simulink model "sim_1"  (R2015b)
settings: Solver=ode23  StartTime=0  StopTime=tstop  FixedStep=1e-3  RelTol=1e-4
undefined symbols (not defined in the file or in its folder): alpha_nc, alpha_nw, currentCoeffMatrix, f, mu, N_freq, Par, phi, S, Sim, U_mean_c, U_mean_w, windCoeffMatrix
libraries: simulink_extras x4, simulink x4
settings Model: Creator=torstebo  LastModifiedBy=ShivJeet
settings SolverCC: MaxConsecutiveMinStep=3  SolverJacobianMethodControl=FullPerturbation  ZeroCrossControl=DisableAll  ZeroCrossAlgorithm=Adaptive
settings DataIOCC: Decimation=10  InitialState=xFinal  LimitDataPoints=off  SaveFormat=StructureWithTime  SaveOutput=off  InspectSignalLogs=on  VisualizeSimOutput=off  SaveTime=off
settings OptimizationCC: AccelVerboseBuild=on
settings DebuggingCC: AlgebraicLoopMsg=error  UnderspecifiedInitializationDetection=Classic  MergeDetectMultiDrivingBlocksExec=none  SolverPrmCheckMsg=warning  StateNameClashWarn=warning
settings HardwareCC: ProdBitPerPointer=32  ProdLargestAtomicFloat=None  ProdIntDivRoundTo=Undefined  ProdEndianess=Unspecified  ProdWordSize=32  ProdHWDeviceType=32-bit Generic
settings GRTTargetCC: GeneratePreprocessorConditionals=Disable all
settings ConfigComp: CovModelRefEnable=Off  CovSFcnEnable=off

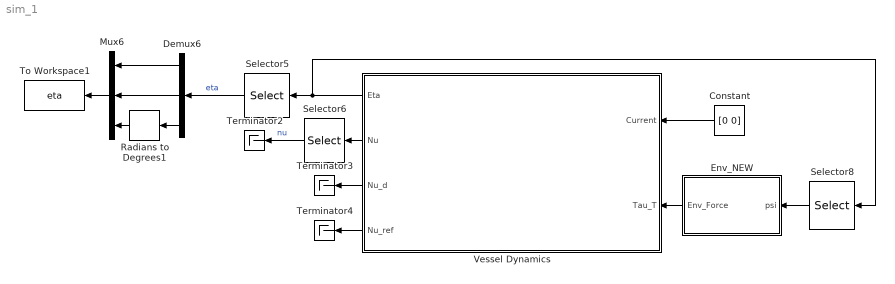
== system sim_1 ==
  Constant : Constant  Value=[0 0]
  Demux6 : Demux  Outputs=3
  Env_NEW : Subsystem
  Mux6 : Mux  Inputs=3
  Radians to Degrees1 : simulink_extras/Transformations/Radians to Degrees
  Selector5 : Selector  InputPortWidth=6  IndexOptions=Index vector (dialog)  Indices=[1 2 6]  OutputSizes=1
  Selector6 : Selector  InputPortWidth=6  IndexOptions=Index vector (dialog)  Indices=[1 2 6]  OutputSizes=1
  Selector8 : Selector  InputPortWidth=6  IndexOptions=Index vector (dialog)  Indices=[6]  OutputSizes=1
  Terminator2 : Terminator
  Terminator3 : Terminator
  Terminator4 : Terminator
  To Workspace1 : ToWorkspace  VariableName=eta  SaveFormat=Timeseries  SampleTime=-1
  Vessel Dynamics : Subsystem
      mask Display:
      | image(imread('Files/supply.jpg'))
      | color('black'); port_label('output', 1, 'eta')
      | color('black'); port_label('output', 2, 'nu')
      | color('black'); port_label('output', 3, 'nu_d')
      | color('black'); port_label('output', 4, 'nu_ref')
      | color('black'); port_label('input', 1, 'nu_c')
      | color('black'); port_label('input', 2, 'tau')
  wires:
  Vessel Dynamics/1(Eta) -> Selector8/1, Selector5/1
  Vessel Dynamics/2(Nu) -> Selector6/1
  Constant/1 -> Vessel Dynamics/1(Current)
  Env_NEW/1(Env_Force) -> Vessel Dynamics/2(Tau_T)
  Selector8/1 -> Env_NEW/1(psi)
  Vessel Dynamics/3(Nu_d) -> Terminator3/1
  Vessel Dynamics/4(Nu_ref) -> Terminator4/1
  Selector5/1 -> Demux6/1  "eta"
  Demux6/3 -> Radians to Degrees1/1
  Radians to Degrees1/1 -> Mux6/3
  Demux6/2 -> Mux6/2
  Demux6/1 -> Mux6/1
  Mux6/1 -> To Workspace1/1
  Selector6/1 -> Terminator2/1  "nu"

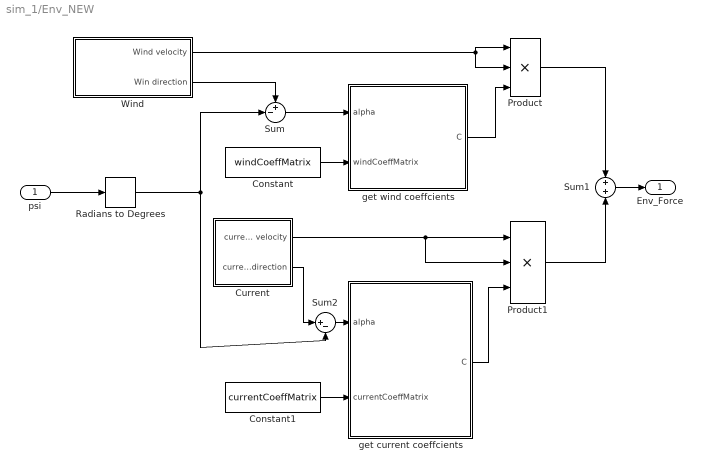
== system sim_1/Env_NEW ==
  psi : Inport
  Constant : Constant  Value=windCoeffMatrix
  Constant1 : Constant  Value=currentCoeffMatrix
  Current : Subsystem
  Product : Product  Inputs=3  RndMeth=Zero
  Product1 : Product  Inputs=3  RndMeth=Zero
  Radians to Degrees : simulink_extras/Transformations/Radians to Degrees
  Sum : Sum  Inputs=+-|
  Sum1 : Sum  Inputs=+|+
  Sum2 : Sum  Inputs=|+-
  Wind : Subsystem
  get current coeffcients : MATLAB Function  TreatAsAtomicUnit=on
  get wind coeffcients : MATLAB Function  TreatAsAtomicUnit=on
  Env_Force : Outport
  wires:
  Wind/1(Wind velocity) -> Product/2, Product/1
  Wind/2(Win direction) -> Sum/1
  psi/1 -> Radians to Degrees/1
  Sum1/1 -> Env_Force/1
  Current/1(current velocity) -> Product1/2, Product1/1
  Radians to Degrees/1 -> Sum/2, Sum2/2
  Current/2(current direction) -> Sum2/1
  Sum2/1 -> get current coeffcients/1(alpha)
  get current coeffcients/1(C) -> Product1/3
  Sum/1 -> get wind coeffcients/1(alpha)
  get wind coeffcients/1(C) -> Product/3
  Product1/1 -> Sum1/2
  Product/1 -> Sum1/1
  Constant/1 -> get wind coeffcients/2(windCoeffMatrix)
  Constant1/1 -> get current coeffcients/2(currentCoeffMatrix)

== system sim_1/Vessel Dynamics ==
  note: VESSEL MODULE
      | Consists of a WF and a LF module, which may be enabled or disabled in the Parameters file.
      | The LF and WFmotion components are written to the workspace for processing, and added for
      | use in the simulator.
  Current : Inport
  Tau_T : Inport  Port=2
  Vessel LF 6DOF : Subsystem
  Eta : Outport
  Nu : Outport  Port=2
  Nu_d : Outport  Port=3
  Nu_ref : Outport  Port=4
  wires:
  Current/1 -> Vessel LF 6DOF/2(Current_NED)
  Tau_T/1 -> Vessel LF 6DOF/1(External forces)  "Tau_T"
  Vessel LF 6DOF/1(Eta) -> Eta/1  "Eta_LF"
  Vessel LF 6DOF/2(Nu) -> Nu/1  "Nu_LF"
  Vessel LF 6DOF/3(Nu_d) -> Nu_d/1
  Vessel LF 6DOF/4(Nu_r) -> Nu_ref/1

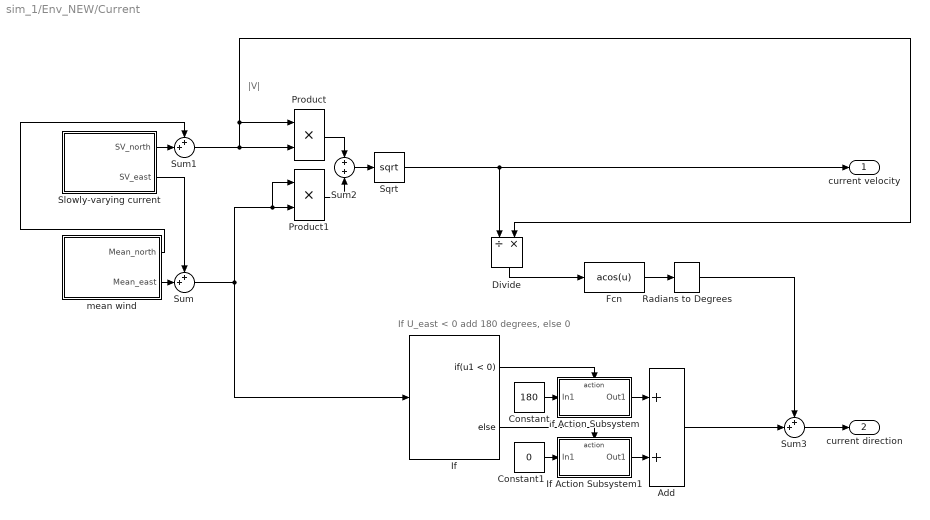
== system sim_1/Env_NEW/Current ==
  note: If U_east < 0 add 180 degrees, else 0
  note: |V|
  Add : Sum
  Constant : Constant  Value=180
  Constant1 : Constant  Value=0
  Divide : Product  Inputs=/*
  Fcn : Fcn  Expr=acos(u)
  "If " : If  IfExpression=u1 < 0
  If Action Subsystem : Subsystem  TreatAsAtomicUnit=on
  If Action Subsystem1 : Subsystem  TreatAsAtomicUnit=on
  Product : Product
  Product1 : Product
  Radians to Degrees : simulink_extras/Transformations/Radians to Degrees
  Slowly-varying current : Subsystem
  Sqrt : Sqrt  SaturateOnIntegerOverflow=on
  Sum : Sum  Inputs=++|
  Sum1 : Sum  Inputs=++|
  Sum2 : Sum  Inputs=+|+
  Sum3 : Sum  Inputs=++|
  mean wind : Subsystem
  current velocity : Outport
  current direction : Outport  Port=2
  wires:
  Slowly-varying current/1(SV_north) -> Sum1/2
  Slowly-varying current/2(SV_east) -> Sum/1
  mean wind/2(Mean_east) -> Sum/2
  Divide/1 -> Fcn/1
  Fcn/1 -> Radians to Degrees/1
  Sum3/1 -> current direction/1
  Radians to Degrees/1 -> Sum3/1
  If Action Subsystem/1(Out1) -> Add/1
  Add/1 -> Sum3/2
  mean wind/1(Mean_north) -> Sum1/1
  Sum1/1 -> Product/2, Product/1, Divide/2
  Sum/1 -> Product1/1, Product1/2, "If "/1
  Product/1 -> Sum2/1
  Product1/1 -> Sum2/2
  Sum2/1 -> Sqrt/1
  Sqrt/1 -> Divide/1, current velocity/1
  Constant/1 -> If Action Subsystem/1(In1)
  "If "/1 -> If Action Subsystem/Action
  "If "/2 -> If Action Subsystem1/Action
  Constant1/1 -> If Action Subsystem1/1(In1)
  If Action Subsystem1/1(Out1) -> Add/2

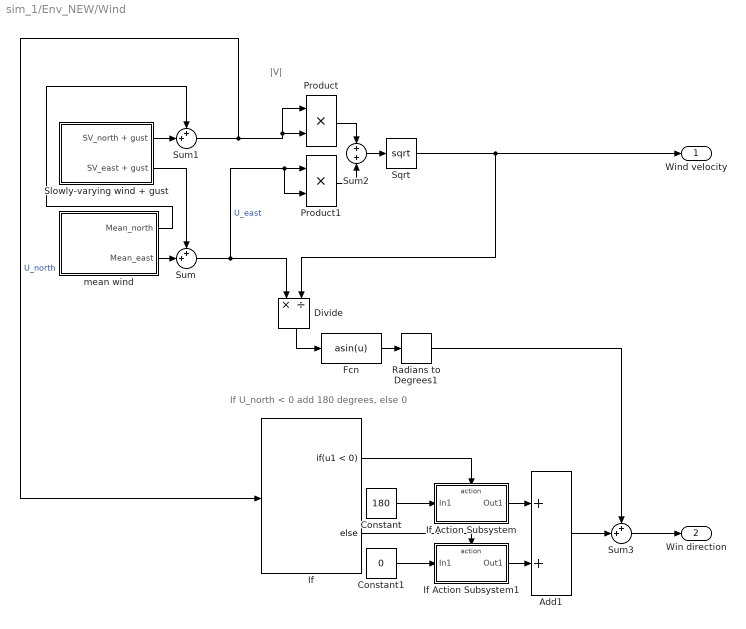
== system sim_1/Env_NEW/Wind ==
  note: |V|
  note: If U_north < 0 add 180 degrees, else 0
  Add1 : Sum
  Constant : Constant  Value=180
  Constant1 : Constant  Value=0
  Divide : Product  Inputs=*/
  Fcn : Fcn  Expr=asin(u)
  If : If  IfExpression=u1 < 0
  If Action Subsystem : Subsystem  TreatAsAtomicUnit=on
  If Action Subsystem1 : Subsystem  TreatAsAtomicUnit=on
  Product : Product
  Product1 : Product
  Radians to Degrees1 : simulink_extras/Transformations/Radians to Degrees
  Slowly-varying wind + gust : Subsystem
  Sqrt : Sqrt  SaturateOnIntegerOverflow=on
  Sum : Sum  Inputs=++|
  Sum1 : Sum  Inputs=++|
  Sum2 : Sum  Inputs=+|+
  Sum3 : Sum  Inputs=++|
  mean wind : Subsystem
  Wind velocity : Outport
  Win direction : Outport  Port=2
  wires:
  Slowly-varying wind + gust/2(SV_east + gust) -> Sum/1
  mean wind/2(Mean_east) -> Sum/2
  Sum1/1 -> Product/1, Product/2, If/1  "U_north"
  Sum/1 -> Product1/2, Product1/1, Divide/1  "U_east"
  Sqrt/1 -> Divide/2, Wind velocity/1
  Slowly-varying wind + gust/1(SV_north + gust) -> Sum1/2
  mean wind/1(Mean_north) -> Sum1/1
  Product/1 -> Sum2/1
  Product1/1 -> Sum2/2
  Sum2/1 -> Sqrt/1
  Divide/1 -> Fcn/1
  Fcn/1 -> Radians to Degrees1/1
  Radians to Degrees1/1 -> Sum3/1
  Add1/1 -> Sum3/2
  Sum3/1 -> Win direction/1
  If Action Subsystem/1(Out1) -> Add1/1
  Constant/1 -> If Action Subsystem/1(In1)
  If/1 -> If Action Subsystem/Action
  If/2 -> If Action Subsystem1/Action
  Constant1/1 -> If Action Subsystem1/1(In1)
  If Action Subsystem1/1(Out1) -> Add1/2

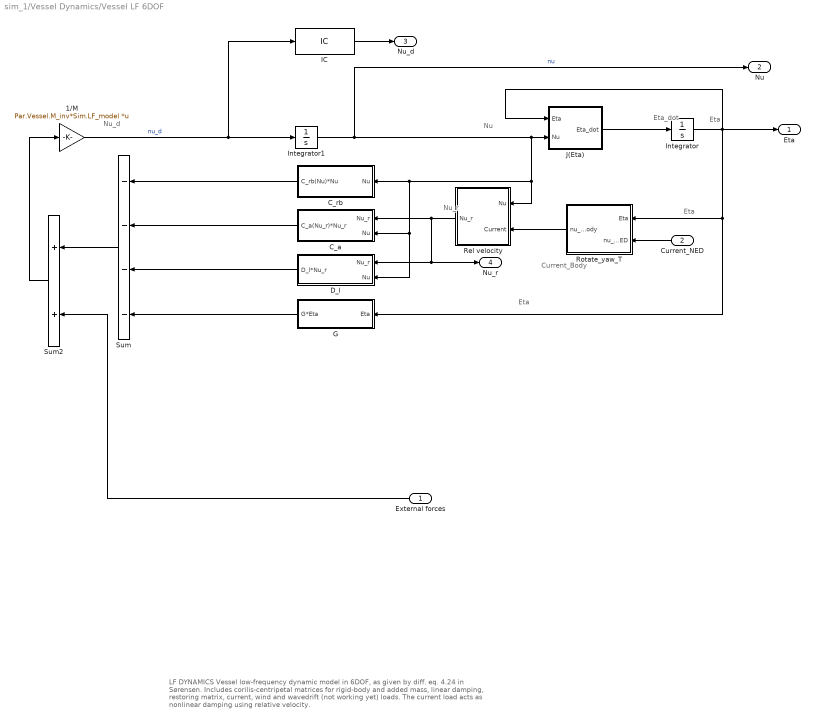
== system sim_1/Vessel Dynamics/Vessel LF 6DOF ==
  note: Nu_d
  note: Nu
  note: Eta
  note: Current_Body
  note: Eta
  note: Nu_r
  note: Eta
  note: LF DYNAMICS
      | Vessel low-frequency dynamic model in 6DOF, as given by diff. eq. 4.24 in Sørensen.
      | Includes corilis-centripetal matrices for rigid-body and added mass, linear damping,
      | restoring matrix, current, wind and wavedrift (not working yet) loads. The current load
      | acts as nonlinear damping using relative velocity.
  note: Eta_dot
  External forces : Inport
  Current_NED : Inport  Port=2
  1/M : Gain  Gain=Par.Vessel.M_inv*Sim.LF_model  Multiplication=Matrix(K*u) (u vector)  SaturateOnIntegerOverflow=on  OutDataTypeStr=Inherit: Same as input  ParamDataTypeStr=Inherit: Same as input
  C_a : Subsystem
  C_rb : Subsystem
  D_l : Subsystem
      settings: MinAlgLoopOccurrences=on
  G : Subsystem
  IC : InitialCondition  Value=Sim.Nu_d_init
  Integrator : Integrator  InitialCondition=Sim.Eta_init
  Integrator1 : Integrator  InitialCondition=Sim.Nu_init
  J(Eta) : Subsystem
  Rel velocity : Subsystem
  Rotate_yaw_T : Subsystem
  Sum : Sum  Inputs=----  SaturateOnIntegerOverflow=on
  Sum2 : Sum  SaturateOnIntegerOverflow=on
  Eta : Outport
  Nu : Outport  Port=2
  Nu_d : Outport  Port=3
  Nu_r : Outport  Port=4
  wires:
  1/M/1 -> IC/1, Integrator1/1  "nu_d"
  J(Eta)/1(Eta_dot) -> Integrator/1
  Integrator/1 -> J(Eta)/1(Eta), Eta/1, Rotate_yaw_T/1(Eta), G/1(Eta)
  Integrator1/1 -> Nu/1, J(Eta)/2(Nu), Rel velocity/1(Nu), C_a/2(Nu), D_l/2(Nu), C_rb/1(Nu)  "nu"
  Current_NED/1 -> Rotate_yaw_T/2(nu_2D_NED)
  Rotate_yaw_T/1(nu_2D_body) -> Rel velocity/2(Current)
  Rel velocity/1(Nu_r) -> D_l/1(Nu_r), Nu_r/1, C_a/1(Nu_r)
  Sum/1 -> Sum2/1
  External forces/1 -> Sum2/2
  Sum2/1 -> 1/M/1
  C_rb/1(C_rb(Nu)*Nu) -> Sum/1
  C_a/1(C_a(Nu_r)*Nu_r) -> Sum/2
  D_l/1(D_l*Nu_r) -> Sum/3
  G/1(G*Eta) -> Sum/4
  IC/1 -> Nu_d/1

== system sim_1/Env_NEW/Current/If Action Subsystem ==
  In1 : Inport
  Action Port : ActionPort  ActionType=then
  Out1 : Outport
  wires:
  In1/1 -> Out1/1

== system sim_1/Env_NEW/Current/If Action Subsystem1 ==
  In1 : Inport
  Action Port : ActionPort  ActionType=else
  Out1 : Outport
  wires:
  In1/1 -> Out1/1

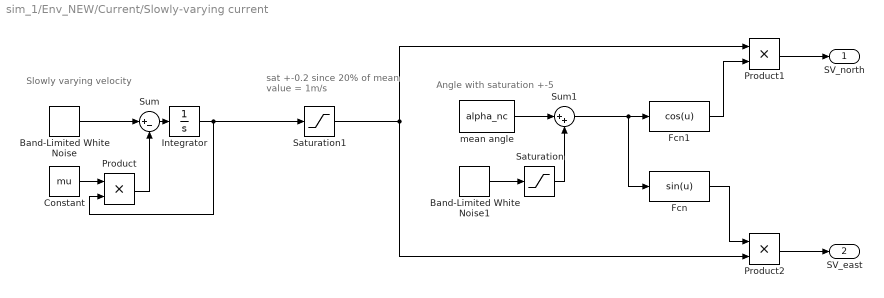
== system sim_1/Env_NEW/Current/Slowly-varying current ==
  note: Angle with saturation +-5
  note: Slowly varying velocity
  note: sat +-0.2 since 20%
      | of mean value = 1m/s
  Band-Limited White Noise : simulink/Sources/Band-Limited White Noise  Cov=[0.00005]  Ts=20  seed=[23343]
  Band-Limited White Noise1 : simulink/Sources/Band-Limited White Noise  Cov=[0.00005]  Ts=20  seed=[23344]
  Constant : Constant  Value=mu
  Fcn : Fcn  Expr=sin(u)
  Fcn1 : Fcn  Expr=cos(u)
  Integrator : Integrator
  Product : Product  RndMeth=Zero
  Product1 : Product  RndMeth=Zero
  Product2 : Product  RndMeth=Zero
  Saturation : Saturate  UpperLimit=(5*pi)/180  LowerLimit=-(5*pi)/180
  Saturation1 : Saturate  UpperLimit=0.2  LowerLimit=-0.2
  Sum : Sum  Inputs=|+-
  Sum1 : Sum  Inputs=|++
  mean angle : Constant  Value=alpha_nc
  SV_north : Outport
  SV_east : Outport  Port=2
  wires:
  Band-Limited White Noise/1 -> Sum/1
  Sum/1 -> Integrator/1
  Integrator/1 -> Product/2, Saturation1/1
  Product/1 -> Sum/2
  Constant/1 -> Product/1
  Fcn1/1 -> Product1/2
  mean angle/1 -> Sum1/1
  Sum1/1 -> Fcn/1, Fcn1/1
  Saturation/1 -> Sum1/2
  Band-Limited White Noise1/1 -> Saturation/1
  Product1/1 -> SV_north/1
  Product2/1 -> SV_east/1
  Saturation1/1 -> Product2/2, Product1/1
  Fcn/1 -> Product2/1

== system sim_1/Env_NEW/Current/mean wind ==
  Constant : Constant  Value=U_mean_c
  Fcn : Fcn  Expr=sin(u)
  Fcn1 : Fcn  Expr=cos(u)
  Product1 : Product  RndMeth=Zero
  Product2 : Product  RndMeth=Zero
  meen wind : Constant  Value=alpha_nc
  Mean_north : Outport
  Mean_east : Outport  Port=2
  wires:
  Constant/1 -> Product1/1, Product2/2
  Fcn1/1 -> Product1/2
  Product1/1 -> Mean_north/1
  Product2/1 -> Mean_east/1
  meen wind/1 -> Fcn/1, Fcn1/1
  Fcn/1 -> Product2/1

== system sim_1/Env_NEW/Wind/If Action Subsystem ==
  In1 : Inport
  Action Port : ActionPort  ActionType=then
  Out1 : Outport
  wires:
  In1/1 -> Out1/1

== system sim_1/Env_NEW/Wind/If Action Subsystem1 ==
  In1 : Inport
  Action Port : ActionPort  ActionType=else
  Out1 : Outport
  wires:
  In1/1 -> Out1/1

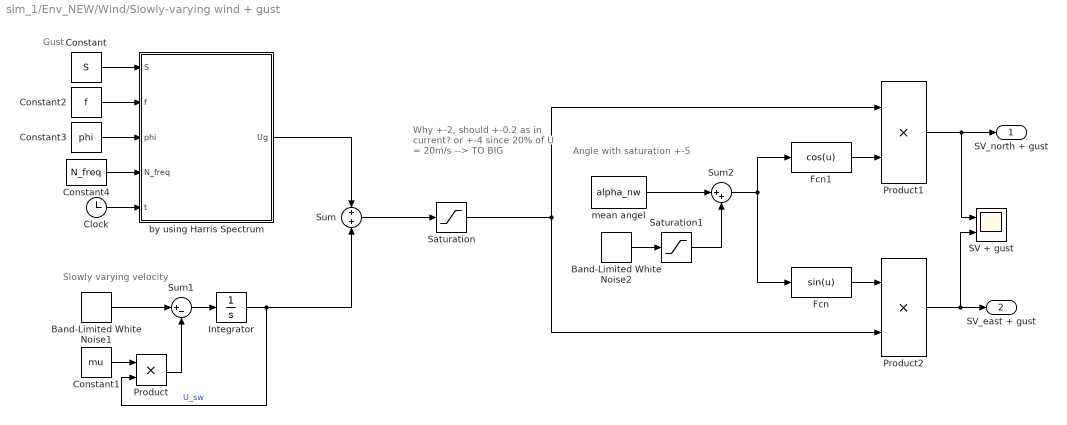
== system sim_1/Env_NEW/Wind/Slowly-varying wind + gust ==
  note: Gust
  note: Slowly varying velocity
  note: Angle with saturation +-5
  note: Why +-2, should
      | +-0.2 as in current?
      | or +-4 since 20% of
      | U = 20m/s --> TO BIG
  Band-Limited White Noise1 : simulink/Sources/Band-Limited White Noise  Cov=[0.005]  Ts=20  seed=[23341]
  Band-Limited White Noise2 : simulink/Sources/Band-Limited White Noise  Cov=[0.005]  Ts=20  seed=[23342]
  Clock : Clock
  Constant : Constant  Value=S
  Constant1 : Constant  Value=mu
  Constant2 : Constant  Value=f
  Constant3 : Constant  Value=phi
  Constant4 : Constant  Value=N_freq
  Fcn : Fcn  Expr=sin(u)
  Fcn1 : Fcn  Expr=cos(u)
  Integrator : Integrator
  Product : Product  RndMeth=Zero
  Product1 : Product  RndMeth=Zero
  Product2 : Product  RndMeth=Zero
  SV + gust : Scope  NumInputPorts=2
  Saturation : Saturate  UpperLimit=2  LowerLimit=-2
  Saturation1 : Saturate  UpperLimit=(5*pi)/180  LowerLimit=-(5*pi)/180
  Sum : Sum  Inputs=+|+
  Sum1 : Sum  Inputs=|+-
  Sum2 : Sum  Inputs=|++
  by using Harris Spectrum : MATLAB Function  TreatAsAtomicUnit=on  SystemSampleTime=1
  mean angel : Constant  Value=alpha_nw
  SV_north + gust : Outport
  SV_east + gust : Outport  Port=2
  wires:
  Fcn1/1 -> Product1/2
  Product1/1 -> SV + gust/1, SV_north + gust/1
  Product2/1 -> SV_east + gust/1, SV + gust/2
  Sum2/1 -> Fcn/1, Fcn1/1
  Integrator/1 -> Sum/2, Product/2  "U_sw"
  Saturation/1 -> Product1/1, Product2/2
  Constant1/1 -> Product/1
  Sum1/1 -> Integrator/1
  Product/1 -> Sum1/2
  Band-Limited White Noise1/1 -> Sum1/1
  mean angel/1 -> Sum2/1
  Saturation1/1 -> Sum2/2
  Band-Limited White Noise2/1 -> Saturation1/1
  Fcn/1 -> Product2/1
  Constant/1 -> by using Harris Spectrum/1(S)
  Constant2/1 -> by using Harris Spectrum/2(f)
  Constant3/1 -> by using Harris Spectrum/3(phi)
  Constant4/1 -> by using Harris Spectrum/4(N_freq)
  Clock/1 -> by using Harris Spectrum/5(t)
  Sum/1 -> Saturation/1
  by using Harris Spectrum/1(Ug) -> Sum/1

== system sim_1/Env_NEW/Wind/mean wind ==
  Constant : Constant  Value=U_mean_w
  Fcn : Fcn  Expr=sin(u)
  Fcn1 : Fcn  Expr=cos(u)
  Product1 : Product  RndMeth=Zero
  Product2 : Product  RndMeth=Zero
  mean wind : Constant  Value=alpha_nw
  Mean_north : Outport
  Mean_east : Outport  Port=2
  wires:
  Constant/1 -> Product2/2, Product1/1
  Fcn1/1 -> Product1/2
  Product1/1 -> Mean_north/1
  mean wind/1 -> Fcn1/1, Fcn/1
  Fcn/1 -> Product2/1
  Product2/1 -> Mean_east/1

== system sim_1/Vessel Dynamics/Vessel LF 6DOF/C_a ==
  note: C_a
      | Coriolis-centripetal added mass force calculation using the S-function m2c_S.
      | This effect can be included/excluded from the Parameters file.
      | A choice of using absolute or relative vessel velocity is also given.
      | OS2002
  Nu_r : Inport
  Nu : Inport  Port=2
  C_a calculation : Subsystem  TreatAsAtomicUnit=on
  Enable Coriolis added mass force : Constant  Value=Sim.C_a
  Sim.Nu_r_C_a : Constant  Value=Sim.Nu_r_C_a
  Switch : Switch  Criteria=u2 > Threshold  SaturateOnIntegerOverflow=on
  C_a(Nu_r)*Nu_r : Outport
  wires:
  C_a calculation/1(F) -> C_a(Nu_r)*Nu_r/1
  Nu_r/1 -> Switch/1
  Nu/1 -> Switch/3
  Sim.Nu_r_C_a/1 -> Switch/2
  Switch/1 -> C_a calculation/1(Nu_r)
  Enable Coriolis added mass force/1 -> C_a calculation/Enable

== system sim_1/Vessel Dynamics/Vessel LF 6DOF/C_rb ==
  note: C_rb
      | Coriolis-centripetal rigid-body force calculation using the S-function m2c_S.
      | This effect can be included/excluded from the Parameters file.
      | OS2002
  Nu : Inport
  C_rb Calculation : Subsystem  TreatAsAtomicUnit=on
  Enable Coriolis added mass force : Constant  Value=Sim.C_rb
  C_rb(Nu)*Nu : Outport
  wires:
  Nu/1 -> C_rb Calculation/1(Nu_r)
  Enable Coriolis added mass force/1 -> C_rb Calculation/Enable
  C_rb Calculation/1(F) -> C_rb(Nu)*Nu/1

== system sim_1/Vessel Dynamics/Vessel LF 6DOF/D_l ==
  note: D_l
      | Linear damping, matrix formulation.
      | This effect can be included/excluded from the Parameters file.
      | A choice of using absolute or relative vessel velocity is also given.
      | OS2002
  Nu_r : Inport
  Nu : Inport  Port=2
  D_l : Gain  Gain=Par.Vessel.DL  Multiplication=Matrix(K*u)  SaturateOnIntegerOverflow=on  OutDataTypeStr=Inherit: Same as input  ParamDataTypeStr=Inherit: Same as input
  Include D_l : Gain  Gain=Sim.D_l  SaturateOnIntegerOverflow=on  OutDataTypeStr=Inherit: Same as input  ParamDataTypeStr=Inherit: Same as input
  Sim.Nu_r_D_l : Constant  Value=Sim.Nu_r_D_l
  Switch : Switch  Criteria=u2 > Threshold  SaturateOnIntegerOverflow=on
  D_l*Nu_r : Outport
  wires:
  D_l/1 -> Include D_l/1
  Include D_l/1 -> D_l*Nu_r/1
  Switch/1 -> D_l/1
  Nu_r/1 -> Switch/1
  Nu/1 -> Switch/3
  Sim.Nu_r_D_l/1 -> Switch/2

== system sim_1/Vessel Dynamics/Vessel LF 6DOF/G ==
  note: G
      | Standard restoring matrix. This effect can
      | be included/excluded from the Parameters file.
      | OS2002
  Eta : Inport
  G : Gain  Gain=Par.Vessel.G  Multiplication=Matrix(K*u)  SaturateOnIntegerOverflow=on  OutDataTypeStr=Inherit: Same as input  ParamDataTypeStr=Inherit: Same as input
  Include G : Gain  Gain=Sim.G  SaturateOnIntegerOverflow=on  OutDataTypeStr=Inherit: Same as input  ParamDataTypeStr=Inherit: Same as input
  G*Eta : Outport
  wires:
  Eta/1 -> G/1
  G/1 -> Include G/1
  Include G/1 -> G*Eta/1

== system sim_1/Vessel Dynamics/Vessel LF 6DOF/J(Eta) ==
  note: Theta
  note: v
  note: omega
  note: J(Eta)
      | Standard 6DOF rotation matrix, as defined by Fossen. Using the two
      | rotation matrices Rnb and Tnb from the gnc Simulink toolbox.
      | OS2002
  Eta : Inport
  Nu : Inport  Port=2
  Mux : Mux  Inputs=2
  Product : Product  Inputs=**  Multiplication=Matrix(*)  SaturateOnIntegerOverflow=on  OutDataTypeStr=Inherit: Same as first input
  Product1 : Product  Inputs=**  Multiplication=Matrix(*)  SaturateOnIntegerOverflow=on  OutDataTypeStr=Inherit: Same as first input
  Rnb_gnc : Subsystem
  Selector : Selector  InputPortWidth=6  IndexOptions=Index vector (dialog)  Indices=[4 5 6]  OutputSizes=1
  Selector1 : Selector  InputPortWidth=6  IndexOptions=Index vector (dialog)  Indices=[1 2 3]  OutputSizes=1
  Selector2 : Selector  InputPortWidth=6  IndexOptions=Index vector (dialog)  Indices=[4 5 6]  OutputSizes=1
  Tnb_gnc : Subsystem
  Eta_dot : Outport
  wires:
  Selector/1 -> Tnb_gnc/1(theta), Rnb_gnc/1(theta)
  Eta/1 -> Selector/1
  Rnb_gnc/1(Rzyx) -> Product/1
  Nu/1 -> Selector1/1, Selector2/1
  Selector1/1 -> Product/2
  Selector2/1 -> Product1/2
  Tnb_gnc/1(T) -> Product1/1
  Product/1 -> Mux/1
  Mux/1 -> Eta_dot/1
  Product1/1 -> Mux/2

== system sim_1/Vessel Dynamics/Vessel LF 6DOF/Rel velocity ==
  note: REL VELOCITY
      | Calculate relative vessel velociy
      | including current.
      | OS2002
  Nu : Inport
  Current : Inport  Port=2
  Mux : Mux  Inputs=2
  Sum : Sum  Inputs=+-  SaturateOnIntegerOverflow=on
  Zeros : Constant  Value=[0 0 0 0]
  Nu_r : Outport
  wires:
  Current/1 -> Mux/1
  Nu/1 -> Sum/1
  Sum/1 -> Nu_r/1
  Mux/1 -> Sum/2
  Zeros/1 -> Mux/2

== system sim_1/Vessel Dynamics/Vessel LF 6DOF/Rotate_yaw_T ==
  note: ROTATE_YAW_T
      | The transposed rotation matrix in yaw, as defined
      | by Fossen. Rotates a velocity or coordinate a positive
      | yaw angle. Corresponds to matlab function  rotate_yaw_T
      | by OS. Uses the gcn Simulink function GNC: "Transposed
      | rotation matrix yaw"
      | OS2002
  Eta : Inport
  nu_2D_NED : Inport  Port=2
  "GNC: \"Transposed rotation matrix yaw\"" : Subsystem
  Mux : Mux  Inputs=2
  Selector : Selector  InputPortWidth=3  IndexOptions=Index vector (dialog)  Indices=[1 2]  OutputSizes=1
  Selector1 : Selector  InputPortWidth=6  IndexOptions=Index vector (dialog)  Indices=6  OutputSizes=1
  psi : Constant  Value=0
  nu_2D_body : Outport
  wires:
  Selector1/1 -> "GNC: \"Transposed rotation matrix yaw\""/1(psi)
  nu_2D_NED/1 -> Mux/1
  psi/1 -> Mux/2
  "GNC: \"Transposed rotation matrix yaw\""/1(R*nu) -> Selector/1
  Selector/1 -> nu_2D_body/1
  Eta/1 -> Selector1/1
  Mux/1 -> "GNC: \"Transposed rotation matrix yaw\""/2(nu)

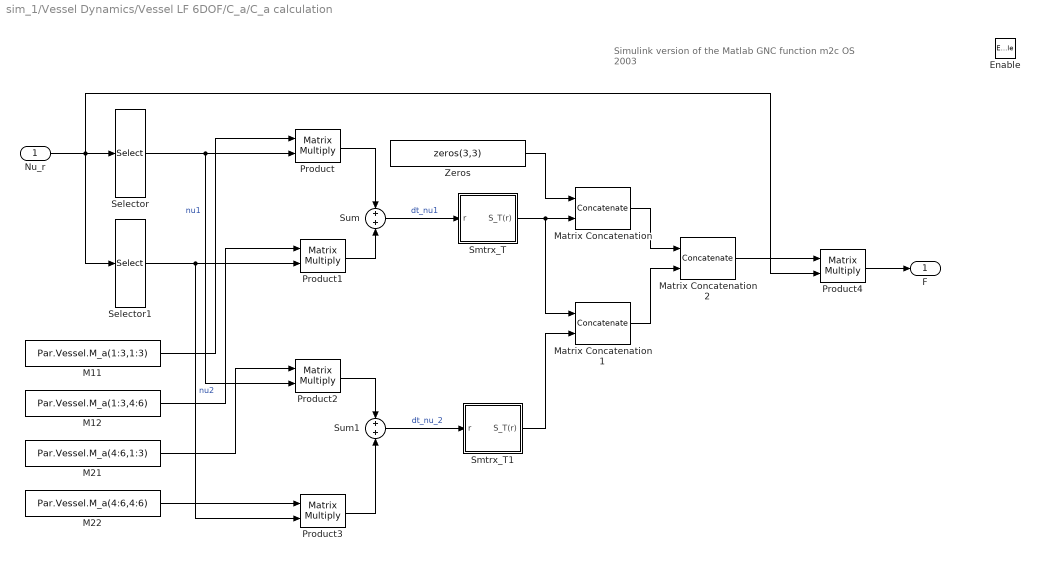
== system sim_1/Vessel Dynamics/Vessel LF 6DOF/C_a/C_a calculation ==
  note: Simulink version of the Matlab GNC function m2c
      | OS 2003
  Nu_r : Inport
  Enable : EnablePort
  M11 : Constant  Value=Par.Vessel.M_a(1:3,1:3)
  M12 : Constant  Value=Par.Vessel.M_a(1:3,4:6)
  M21 : Constant  Value=Par.Vessel.M_a(4:6,1:3)
  M22 : Constant  Value=Par.Vessel.M_a(4:6,4:6)
  Matrix Concatenation : Concatenate  Mode=Multidimensional array  ConcatenateDimension=2
  Matrix Concatenation1 : Concatenate  Mode=Multidimensional array  ConcatenateDimension=2
  Matrix Concatenation2 : Concatenate  Mode=Multidimensional array
  Product{,1..4} (5 alike) : Product  Multiplication=Matrix(*)  SaturateOnIntegerOverflow=on  OutDataTypeStr=Inherit: Same as first input
  Selector : Selector  InputPortWidth=6  IndexOptions=Index vector (dialog)  Indices=[1:3]  OutputSizes=1
  Selector1 : Selector  InputPortWidth=6  IndexOptions=Index vector (dialog)  Indices=[4:6]  OutputSizes=1
  Smtrx_T : Subsystem
  Smtrx_T1 : Subsystem
  Sum : Sum  Inputs=+|+  SaturateOnIntegerOverflow=on
  Sum1 : Sum  Inputs=+|+  SaturateOnIntegerOverflow=on
  Zeros : Constant  Value=zeros(3,3)
  F : Outport
  wires:
  Nu_r/1 -> Selector/1, Selector1/1, Product4/2
  Product/1 -> Sum/1
  Product1/1 -> Sum/2
  Product2/1 -> Sum1/1
  Product3/1 -> Sum1/2
  Sum/1 -> Smtrx_T/1(r)  "dt_nu1"
  Sum1/1 -> Smtrx_T1/1(r)  "dt_nu_2"
  Zeros/1 -> Matrix Concatenation/1
  Smtrx_T/1(S_T(r)) -> Matrix Concatenation/2, Matrix Concatenation1/1
  Smtrx_T1/1(S_T(r)) -> Matrix Concatenation1/2
  Matrix Concatenation/1 -> Matrix Concatenation2/1
  Matrix Concatenation1/1 -> Matrix Concatenation2/2
  Product4/1 -> F/1
  Selector/1 -> Product/2, Product2/2  "nu1"
  Selector1/1 -> Product1/2, Product3/2  "nu2"
  M11/1 -> Product/1
  M12/1 -> Product1/1
  M22/1 -> Product3/1
  M21/1 -> Product2/1
  Matrix Concatenation2/1 -> Product4/1

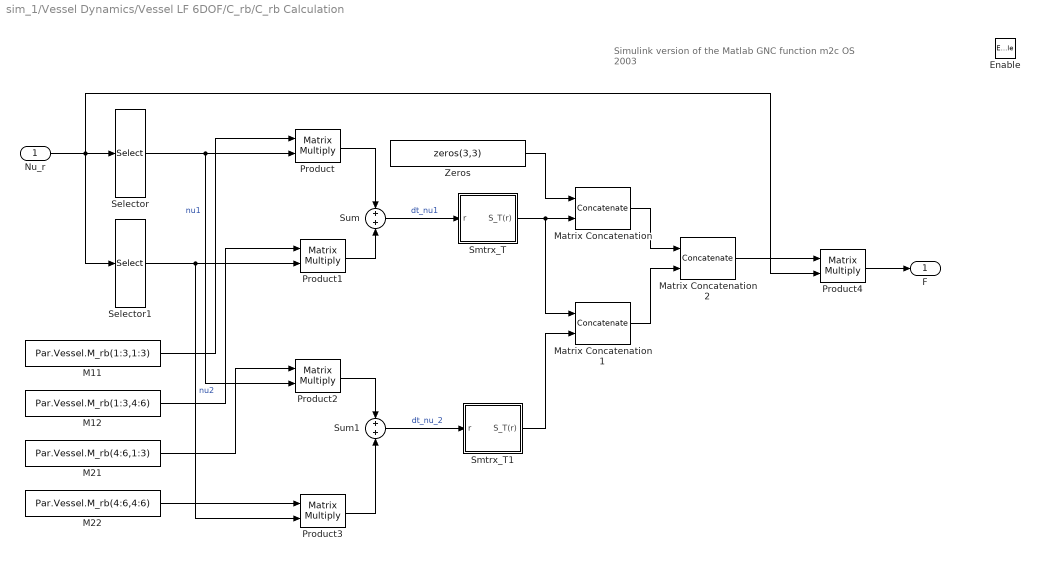
== system sim_1/Vessel Dynamics/Vessel LF 6DOF/C_rb/C_rb Calculation ==
  note: Simulink version of the Matlab GNC function m2c
      | OS 2003
  Nu_r : Inport
  Enable : EnablePort
  M11 : Constant  Value=Par.Vessel.M_rb(1:3,1:3)
  M12 : Constant  Value=Par.Vessel.M_rb(1:3,4:6)
  M21 : Constant  Value=Par.Vessel.M_rb(4:6,1:3)
  M22 : Constant  Value=Par.Vessel.M_rb(4:6,4:6)
  Matrix Concatenation : Concatenate  Mode=Multidimensional array  ConcatenateDimension=2
  Matrix Concatenation1 : Concatenate  Mode=Multidimensional array  ConcatenateDimension=2
  Matrix Concatenation2 : Concatenate  Mode=Multidimensional array
  Product{,1..4} (5 alike) : Product  Multiplication=Matrix(*)  SaturateOnIntegerOverflow=on  OutDataTypeStr=Inherit: Same as first input
  Selector : Selector  InputPortWidth=6  IndexOptions=Index vector (dialog)  Indices=[1:3]  OutputSizes=1
  Selector1 : Selector  InputPortWidth=6  IndexOptions=Index vector (dialog)  Indices=[4:6]  OutputSizes=1
  Smtrx_T : Subsystem
  Smtrx_T1 : Subsystem
  Sum : Sum  Inputs=+|+  SaturateOnIntegerOverflow=on
  Sum1 : Sum  Inputs=+|+  SaturateOnIntegerOverflow=on
  Zeros : Constant  Value=zeros(3,3)
  F : Outport
  wires:
  Nu_r/1 -> Selector/1, Selector1/1, Product4/2
  Product/1 -> Sum/1
  Product1/1 -> Sum/2
  Product2/1 -> Sum1/1
  Product3/1 -> Sum1/2
  Sum/1 -> Smtrx_T/1(r)  "dt_nu1"
  Sum1/1 -> Smtrx_T1/1(r)  "dt_nu_2"
  Zeros/1 -> Matrix Concatenation/1
  Smtrx_T/1(S_T(r)) -> Matrix Concatenation/2, Matrix Concatenation1/1
  Smtrx_T1/1(S_T(r)) -> Matrix Concatenation1/2
  Matrix Concatenation/1 -> Matrix Concatenation2/1
  Matrix Concatenation1/1 -> Matrix Concatenation2/2
  Product4/1 -> F/1
  Selector/1 -> Product/2, Product2/2  "nu1"
  Selector1/1 -> Product1/2, Product3/2  "nu2"
  M11/1 -> Product/1
  M12/1 -> Product1/1
  M22/1 -> Product3/1
  M21/1 -> Product2/1
  Matrix Concatenation2/1 -> Product4/1

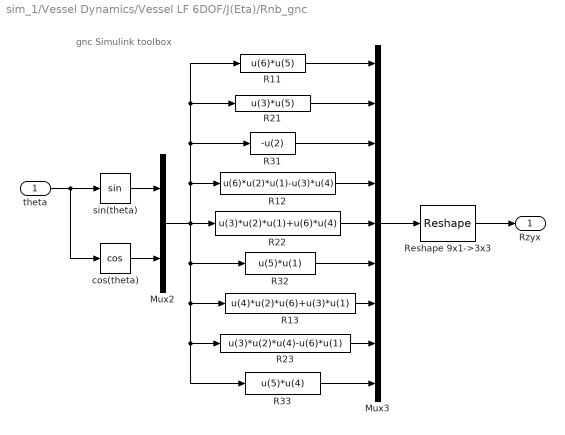
== system sim_1/Vessel Dynamics/Vessel LF 6DOF/J(Eta)/Rnb_gnc ==
  note: gnc Simulink toolbox
  theta : Inport
  Mux2 : Mux  Inputs=2
  Mux3 : Mux  Inputs=9
  R11 : Fcn  Expr=u(6)*u(5)
  R12 : Fcn  Expr=u(6)*u(2)*u(1)-u(3)*u(4)
  R13 : Fcn  Expr=u(4)*u(2)*u(6)+u(3)*u(1)
  "R21 " : Fcn  Expr=u(3)*u(5)
  R22 : Fcn  Expr=u(3)*u(2)*u(1)+u(6)*u(4)
  R23 : Fcn  Expr=u(3)*u(2)*u(4)-u(6)*u(1)
  "R31 " : Fcn  Expr=-u(2)
  R32 : Fcn  Expr=u(5)*u(1)
  R33 : Fcn  Expr=u(5)*u(4)
  Reshape 9x1->3x3 : Reshape  OutputDimensionality=Customize  OutputDimensions=[3,3]
  cos(theta) : Trigonometry  Operator=cos
  sin(theta) : Trigonometry
  Rzyx : Outport  InitialOutput=0
  wires:
  R11/1 -> Mux3/1
  Mux3/1 -> Reshape 9x1->3x3/1
  Reshape 9x1->3x3/1 -> Rzyx/1
  sin(theta)/1 -> Mux2/1
  cos(theta)/1 -> Mux2/2
  theta/1 -> cos(theta)/1, sin(theta)/1
  Mux2/1 -> R32/1, R13/1, R33/1, R23/1, R22/1, "R31 "/1, R11/1, "R21 "/1, R12/1
  R23/1 -> Mux3/8
  R13/1 -> Mux3/7
  R22/1 -> Mux3/5
  R12/1 -> Mux3/4
  "R31 "/1 -> Mux3/3
  "R21 "/1 -> Mux3/2
  R32/1 -> Mux3/6
  R33/1 -> Mux3/9

== system sim_1/Vessel Dynamics/Vessel LF 6DOF/J(Eta)/Tnb_gnc ==
  note: gnc Simulink toolbox
  theta : Inport
  Constant : Constant
  "Constant " : Constant  Value=0
  Mux2 : Mux  Inputs=9
  Reshape 9x1->3x3 : Reshape  OutputDimensionality=Customize  OutputDimensions=[3,3]
  "T21 " : Fcn  Expr=sin(u(1))*tan(u(2))
  T22 : Fcn  Expr=cos(u(1))
  T23 : Fcn  Expr=sin(u(1))/cos(u(2))
  "T31 " : Fcn  Expr=cos(u(1))*tan(u(2))
  T32 : Fcn  Expr=-sin(u(1))
  T33 : Fcn  Expr=cos(u(1))/cos(u(2))
  T : Outport  InitialOutput=0
  wires:
  Constant/1 -> Mux2/1
  Mux2/1 -> Reshape 9x1->3x3/1
  Reshape 9x1->3x3/1 -> T/1
  theta/1 -> "T21 "/1, T22/1, "T31 "/1, T32/1, T33/1, T23/1
  T23/1 -> Mux2/6
  T22/1 -> Mux2/5
  T33/1 -> Mux2/9
  "Constant "/1 -> Mux2/2, Mux2/3
  "T21 "/1 -> Mux2/4
  "T31 "/1 -> Mux2/7
  T32/1 -> Mux2/8

== system sim_1/Vessel Dynamics/Vessel LF 6DOF/Rotate_yaw_T/GNC: "Transposed rotation matrix yaw" ==
  note: GNC: "Transposed
      | rotation matrix yaw"
  psi : Inport
  nu : Inport  Port=2  PortDimensions=3
  Fcn : Fcn  Expr=cos(u(1))*u(2)+sin(u(1))*u(3)
  Fcn1 : Fcn  Expr=-sin(u(1))*u(2)+cos(u(1))*u(3)
  Fcn2 : Fcn  Expr=u(4)
  Mux2 : Mux  Inputs=2
  Mux3 : Mux  Inputs=3
  R*nu : Outport
  wires:
  Mux2/1 -> Fcn1/1, Fcn/1, Fcn2/1
  Fcn/1 -> Mux3/1  "x_dot"
  Fcn1/1 -> Mux3/2  "y_dot"
  Fcn2/1 -> Mux3/3  "psi_dot"
  Mux3/1 -> R*nu/1  "eta_dot"
  psi/1 -> Mux2/1
  nu/1 -> Mux2/2

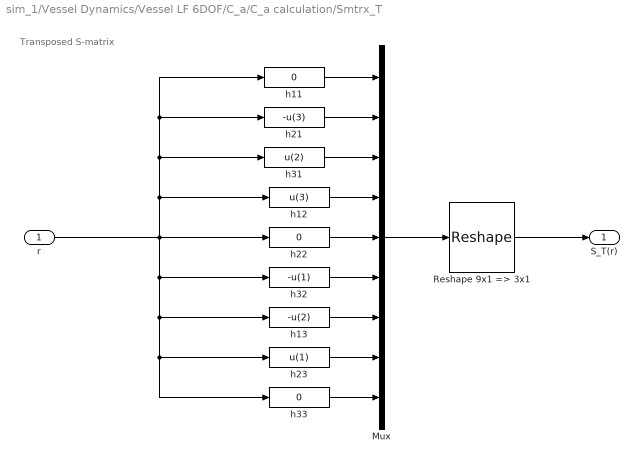
== system sim_1/Vessel Dynamics/Vessel LF 6DOF/C_a/C_a calculation/Smtrx_T ==
  note: Transposed S-matrix
  r : Inport
  Mux : Mux  Inputs=9
  Reshape 9x1 => 3x1 : Reshape  OutputDimensionality=Customize  OutputDimensions=[3,3]
  h11 : Fcn  Expr=0
  h12 : Fcn  Expr=u(3)
  h13 : Fcn  Expr=-u(2)
  h21 : Fcn  Expr=-u(3)
  h22 : Fcn  Expr=0
  h23 : Fcn  Expr=u(1)
  h31 : Fcn  Expr=u(2)
  h32 : Fcn  Expr=-u(1)
  h33 : Fcn  Expr=0
  S_T(r) : Outport
  wires:
  r/1 -> h33/1, h23/1, h13/1, h32/1, h22/1, h12/1, h21/1, h11/1, h31/1
  h33/1 -> Mux/9
  h23/1 -> Mux/8
  h13/1 -> Mux/7
  h32/1 -> Mux/6
  h22/1 -> Mux/5
  h12/1 -> Mux/4
  h31/1 -> Mux/3
  h21/1 -> Mux/2
  h11/1 -> Mux/1
  Mux/1 -> Reshape 9x1 => 3x1/1
  Reshape 9x1 => 3x1/1 -> S_T(r)/1

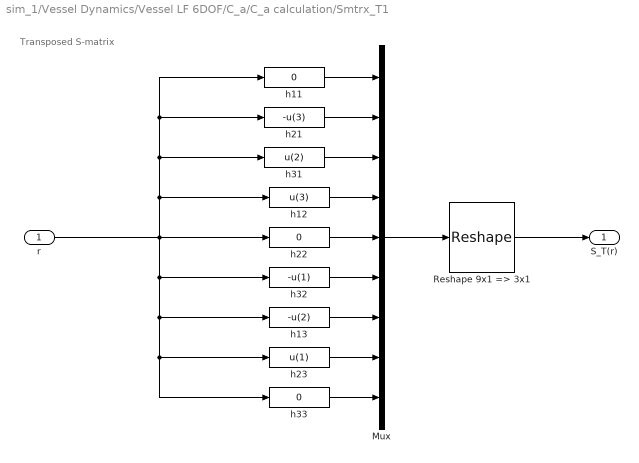
== system sim_1/Vessel Dynamics/Vessel LF 6DOF/C_a/C_a calculation/Smtrx_T1 ==
  note: Transposed S-matrix
  r : Inport
  Mux : Mux  Inputs=9
  Reshape 9x1 => 3x1 : Reshape  OutputDimensionality=Customize  OutputDimensions=[3,3]
  h11 : Fcn  Expr=0
  h12 : Fcn  Expr=u(3)
  h13 : Fcn  Expr=-u(2)
  h21 : Fcn  Expr=-u(3)
  h22 : Fcn  Expr=0
  h23 : Fcn  Expr=u(1)
  h31 : Fcn  Expr=u(2)
  h32 : Fcn  Expr=-u(1)
  h33 : Fcn  Expr=0
  S_T(r) : Outport
  wires:
  Reshape 9x1 => 3x1/1 -> S_T(r)/1
  Mux/1 -> Reshape 9x1 => 3x1/1
  h11/1 -> Mux/1
  h21/1 -> Mux/2
  h31/1 -> Mux/3
  h12/1 -> Mux/4
  h22/1 -> Mux/5
  h32/1 -> Mux/6
  h13/1 -> Mux/7
  h23/1 -> Mux/8
  h33/1 -> Mux/9
  r/1 -> h31/1, h11/1, h21/1, h12/1, h22/1, h32/1, h13/1, h23/1, h33/1

== system sim_1/Vessel Dynamics/Vessel LF 6DOF/C_rb/C_rb Calculation/Smtrx_T ==
  note: Transposed S-matrix
  r : Inport
  Mux : Mux  Inputs=9
  Reshape 9x1 => 3x1 : Reshape  OutputDimensionality=Customize  OutputDimensions=[3,3]
  h11 : Fcn  Expr=0
  h12 : Fcn  Expr=u(3)
  h13 : Fcn  Expr=-u(2)
  h21 : Fcn  Expr=-u(3)
  h22 : Fcn  Expr=0
  h23 : Fcn  Expr=u(1)
  h31 : Fcn  Expr=u(2)
  h32 : Fcn  Expr=-u(1)
  h33 : Fcn  Expr=0
  S_T(r) : Outport
  wires:
  r/1 -> h22/1, h12/1, h21/1, h11/1, h31/1, h33/1, h23/1, h13/1, h32/1
  h33/1 -> Mux/9
  h23/1 -> Mux/8
  h13/1 -> Mux/7
  h32/1 -> Mux/6
  h22/1 -> Mux/5
  h12/1 -> Mux/4
  h31/1 -> Mux/3
  h21/1 -> Mux/2
  h11/1 -> Mux/1
  Mux/1 -> Reshape 9x1 => 3x1/1
  Reshape 9x1 => 3x1/1 -> S_T(r)/1

== system sim_1/Vessel Dynamics/Vessel LF 6DOF/C_rb/C_rb Calculation/Smtrx_T1 ==
  note: Transposed S-matrix
  r : Inport
  Mux : Mux  Inputs=9
  Reshape 9x1 => 3x1 : Reshape  OutputDimensionality=Customize  OutputDimensions=[3,3]
  h11 : Fcn  Expr=0
  h12 : Fcn  Expr=u(3)
  h13 : Fcn  Expr=-u(2)
  h21 : Fcn  Expr=-u(3)
  h22 : Fcn  Expr=0
  h23 : Fcn  Expr=u(1)
  h31 : Fcn  Expr=u(2)
  h32 : Fcn  Expr=-u(1)
  h33 : Fcn  Expr=0
  S_T(r) : Outport
  wires:
  Reshape 9x1 => 3x1/1 -> S_T(r)/1
  Mux/1 -> Reshape 9x1 => 3x1/1
  h11/1 -> Mux/1
  h21/1 -> Mux/2
  h31/1 -> Mux/3
  h12/1 -> Mux/4
  h22/1 -> Mux/5
  h32/1 -> Mux/6
  h13/1 -> Mux/7
  h23/1 -> Mux/8
  h33/1 -> Mux/9
  r/1 -> h31/1, h11/1, h21/1, h12/1, h22/1, h32/1, h13/1, h23/1, h33/1

== matlab function sim_1/Env_NEW/Wind/Slowly-varying wind + gust/by using Harris Spectrum ==
  data: S input; Ug output; f input; phi input; N_freq input; t input
function Ug = fcn(S, f, phi, N_freq, t)
Ug = 0; % dummy value due to Ug first defined in for-loop
for i = 1:N_freq
    Ug = Ug + sqrt(2*S(i)*(f(2)-f(1))) * cos(2*pi*f(i)*t + phi(i));
end
end

== matlab function sim_1/Env_NEW/get current coeffcients ==
  data: alpha input; C output; currentCoeffMatrix input
function C   = CurrentCoefficients( alpha, currentCoeffMatrix )
% Initialization of the return parameter
C=zeros(6,1);

while alpha > 360
    alpha = alpha - 360;
end

while alpha < 0
    alpha = alpha + 360;
end

alpha_mod = mod(alpha,10);
avrundet_alpha = alpha - alpha_mod;
index = avrundet_alpha/10+1;

C1 = currentCoeffMatrix(index,:)';
C2 = currentCoeffMatrix(index+1,:)';

for i = 1:6
    diff = C2(i)-C1(i);
    point = (diff/10)*alpha_mod;
    C(i) = C1(i)+point;
end

end

== matlab function sim_1/Env_NEW/get wind coeffcients ==
  data: alpha input; C output; windCoeffMatrix input
function C   = WindCoeffcients(alpha, windCoeffMatrix)
% Initialization of the return parameter
C=zeros(6,1);

while alpha > 360
    alpha = alpha - 360;
end

while alpha < 0
    alpha = alpha + 360;
end

alpha_mod = mod(alpha,10);
avrundet_alpha = alpha - alpha_mod;
index = avrundet_alpha/10+1;

C1 = windCoeffMatrix(index,:)';
C2 = windCoeffMatrix(index+1,:)';

for i = 1:6
    diff = C2(i)-C1(i);
    point = (diff/10)*alpha_mod;
    C(i) = C1(i)+point;
end

end
